simulink model "AcO_Ctrl_Geometric_headless_R2016a"  (R2016a)
settings: Solver=FixedStepDiscrete  StartTime=0.0  StopTime=simulation_duration  FixedStep=Ts  RelTol=1e-3
values from neighbouring files (symbols this model uses):
  M1_BeMo_d = zeros(7,M1_n_mode)    [AcO_Ctrl_headless_cfg.m]    (also in agws_cfg.m = 1e-6*bsxfun(@times,randn(7,M1_n_mode),scale); agws_fastTT_cfg.m = 1e-6*bsxfun(@times,randn(7,M1_n_mode),scale))
  M1_RiBo_d = zeros(7,6)    [AcO_Ctrl_headless_cfg.m]    (also in agws_cfg.m = [M1_Txyz0 M1_Rxyz0]; agws_fastTT_cfg.m = [M1_Txyz0 M1_Rxyz0])
  M2_RiBo_d = zeros(7,6)    [AcO_Ctrl_headless_cfg.m]    (also in agws_cfg.m = [M2_Txyz0 M2_Rxyz0]; agws_fastTT_cfg.m = [M2_Txyz0 M2_Rxyz0])
  Ts = 1/fs    (= 0.002)    [AcO_Ctrl_headless_cfg.m]    (also in agws_fastTT_cfg.m = 0.005)
undefined symbols (not defined in the file or in its folder): Az_C, CG2Hp, CG2Hp_S7, El_C, Fsmm, GIR_C, Hp2CG_f, Hp2CG_f_S7, HPdtf, HpK, KM2, M2_actdyn, M2_CG2Hp, M_LOS, MIMO_C, PTT2act, PTT2act_even, Q, sysd, TT2act, TT2act_even
undefined symbols (not defined in the file): on_axis_src_outputs
libraries: CEO x2
(part 6 of 6)

== system AcO_Ctrl_Geometric_headless_R2016a/Structural Dynamics V3.3/Structural Dynamics V3.5.3/Structural Dynamics Plus CL Az El M1 force/M1 Force Control/ControlM1S1/MIMO Controller ==
  In1 : Inport
  Demux1 : Demux  Outputs=6
  Gain{,1..5} (6 alike) : Gain
  Mux1 : Mux  Inputs=6
  R1 Controller : DiscreteTransferFcn  Numerator=MIMO_C(4,4).num{1}  Denominator=MIMO_C(4,4).den{1}
  R2 Controller : DiscreteTransferFcn  Numerator=MIMO_C(5,5).num{1}  Denominator=MIMO_C(5,5).den{1}
  R3 Controller : DiscreteTransferFcn  Numerator=MIMO_C(6,6).num{1}  Denominator=MIMO_C(6,6).den{1}
  T1 Controller : DiscreteTransferFcn  Numerator=MIMO_C(1,1).num{1}  Denominator=MIMO_C(1,1).den{1}
  T2 Controller : DiscreteTransferFcn  Numerator=MIMO_C(2,2).num{1}  Denominator=MIMO_C(2,2).den{1}
  T3 Controller : DiscreteTransferFcn  Numerator=MIMO_C(3,3).num{1}  Denominator=MIMO_C(3,3).den{1}
  Out1 : Outport
  wires:
  Gain5/1 -> T3 Controller/1
  Gain4/1 -> R3 Controller/1
  Gain3/1 -> R2 Controller/1
  Gain2/1 -> R1 Controller/1
  Gain1/1 -> T2 Controller/1
  Gain/1 -> T1 Controller/1
  Mux1/1 -> Out1/1
  T1 Controller/1 -> Mux1/1
  T2 Controller/1 -> Mux1/2
  T3 Controller/1 -> Mux1/3
  R1 Controller/1 -> Mux1/4
  R2 Controller/1 -> Mux1/5
  R3 Controller/1 -> Mux1/6
  Demux1/6 -> Gain4/1
  Demux1/5 -> Gain3/1
  Demux1/4 -> Gain2/1
  Demux1/3 -> Gain5/1
  Demux1/2 -> Gain1/1
  Demux1/1 -> Gain/1
  In1/1 -> Demux1/1

== system AcO_Ctrl_Geometric_headless_R2016a/Structural Dynamics V3.3/Structural Dynamics V3.5.3/Structural Dynamics Plus CL Az El M1 force/M1 Force Control/ControlM1S2/MIMO Controller ==
  In1 : Inport
  Demux1 : Demux  Outputs=6
  Gain{,1..5} (6 alike) : Gain
  Mux1 : Mux  Inputs=6
  R1 Controller : DiscreteTransferFcn  Numerator=MIMO_C(4,4).num{1}  Denominator=MIMO_C(4,4).den{1}
  R2 Controller : DiscreteTransferFcn  Numerator=MIMO_C(5,5).num{1}  Denominator=MIMO_C(5,5).den{1}
  R3 Controller : DiscreteTransferFcn  Numerator=MIMO_C(6,6).num{1}  Denominator=MIMO_C(6,6).den{1}
  T1 Controller : DiscreteTransferFcn  Numerator=MIMO_C(1,1).num{1}  Denominator=MIMO_C(1,1).den{1}
  T2 Controller : DiscreteTransferFcn  Numerator=MIMO_C(2,2).num{1}  Denominator=MIMO_C(2,2).den{1}
  T3 Controller : DiscreteTransferFcn  Numerator=MIMO_C(3,3).num{1}  Denominator=MIMO_C(3,3).den{1}
  Out1 : Outport
  wires:
  In1/1 -> Demux1/1
  Demux1/1 -> Gain/1
  Demux1/2 -> Gain1/1
  Demux1/3 -> Gain5/1
  Demux1/4 -> Gain2/1
  Demux1/5 -> Gain3/1
  Demux1/6 -> Gain4/1
  R3 Controller/1 -> Mux1/6
  R2 Controller/1 -> Mux1/5
  R1 Controller/1 -> Mux1/4
  T3 Controller/1 -> Mux1/3
  T2 Controller/1 -> Mux1/2
  T1 Controller/1 -> Mux1/1
  Mux1/1 -> Out1/1
  Gain/1 -> T1 Controller/1
  Gain1/1 -> T2 Controller/1
  Gain2/1 -> R1 Controller/1
  Gain3/1 -> R2 Controller/1
  Gain4/1 -> R3 Controller/1
  Gain5/1 -> T3 Controller/1

== system AcO_Ctrl_Geometric_headless_R2016a/Structural Dynamics V3.3/Structural Dynamics V3.5.3/Structural Dynamics Plus CL Az El M1 force/M1 Force Control/ControlM1S3/MIMO Controller ==
  In1 : Inport
  Demux1 : Demux  Outputs=6
  Gain{,1..5} (6 alike) : Gain
  Mux1 : Mux  Inputs=6
  R1 Controller : DiscreteTransferFcn  Numerator=MIMO_C(4,4).num{1}  Denominator=MIMO_C(4,4).den{1}
  R2 Controller : DiscreteTransferFcn  Numerator=MIMO_C(5,5).num{1}  Denominator=MIMO_C(5,5).den{1}
  R3 Controller : DiscreteTransferFcn  Numerator=MIMO_C(6,6).num{1}  Denominator=MIMO_C(6,6).den{1}
  T1 Controller : DiscreteTransferFcn  Numerator=MIMO_C(1,1).num{1}  Denominator=MIMO_C(1,1).den{1}
  T2 Controller : DiscreteTransferFcn  Numerator=MIMO_C(2,2).num{1}  Denominator=MIMO_C(2,2).den{1}
  T3 Controller : DiscreteTransferFcn  Numerator=MIMO_C(3,3).num{1}  Denominator=MIMO_C(3,3).den{1}
  Out1 : Outport
  wires:
  Gain5/1 -> T3 Controller/1
  Gain4/1 -> R3 Controller/1
  Gain3/1 -> R2 Controller/1
  Gain2/1 -> R1 Controller/1
  Gain1/1 -> T2 Controller/1
  Gain/1 -> T1 Controller/1
  Mux1/1 -> Out1/1
  T1 Controller/1 -> Mux1/1
  T2 Controller/1 -> Mux1/2
  T3 Controller/1 -> Mux1/3
  R1 Controller/1 -> Mux1/4
  R2 Controller/1 -> Mux1/5
  R3 Controller/1 -> Mux1/6
  Demux1/6 -> Gain4/1
  Demux1/5 -> Gain3/1
  Demux1/4 -> Gain2/1
  Demux1/3 -> Gain5/1
  Demux1/2 -> Gain1/1
  Demux1/1 -> Gain/1
  In1/1 -> Demux1/1

== system AcO_Ctrl_Geometric_headless_R2016a/Structural Dynamics V3.3/Structural Dynamics V3.5.3/Structural Dynamics Plus CL Az El M1 force/M1 Force Control/ControlM1S4/MIMO Controller ==
  In1 : Inport
  Demux1 : Demux  Outputs=6
  Gain{,1..5} (6 alike) : Gain
  Mux1 : Mux  Inputs=6
  R1 Controller : DiscreteTransferFcn  Numerator=MIMO_C(4,4).num{1}  Denominator=MIMO_C(4,4).den{1}
  R2 Controller : DiscreteTransferFcn  Numerator=MIMO_C(5,5).num{1}  Denominator=MIMO_C(5,5).den{1}
  R3 Controller : DiscreteTransferFcn  Numerator=MIMO_C(6,6).num{1}  Denominator=MIMO_C(6,6).den{1}
  T1 Controller : DiscreteTransferFcn  Numerator=MIMO_C(1,1).num{1}  Denominator=MIMO_C(1,1).den{1}
  T2 Controller : DiscreteTransferFcn  Numerator=MIMO_C(2,2).num{1}  Denominator=MIMO_C(2,2).den{1}
  T3 Controller : DiscreteTransferFcn  Numerator=MIMO_C(3,3).num{1}  Denominator=MIMO_C(3,3).den{1}
  Out1 : Outport
  wires:
  In1/1 -> Demux1/1
  Demux1/1 -> Gain/1
  Demux1/2 -> Gain1/1
  Demux1/3 -> Gain5/1
  Demux1/4 -> Gain2/1
  Demux1/5 -> Gain3/1
  Demux1/6 -> Gain4/1
  R3 Controller/1 -> Mux1/6
  R2 Controller/1 -> Mux1/5
  R1 Controller/1 -> Mux1/4
  T3 Controller/1 -> Mux1/3
  T2 Controller/1 -> Mux1/2
  T1 Controller/1 -> Mux1/1
  Mux1/1 -> Out1/1
  Gain/1 -> T1 Controller/1
  Gain1/1 -> T2 Controller/1
  Gain2/1 -> R1 Controller/1
  Gain3/1 -> R2 Controller/1
  Gain4/1 -> R3 Controller/1
  Gain5/1 -> T3 Controller/1

== system AcO_Ctrl_Geometric_headless_R2016a/Structural Dynamics V3.3/Structural Dynamics V3.5.3/Structural Dynamics Plus CL Az El M1 force/M1 Force Control/ControlM1S5/MIMO Controller ==
  In1 : Inport
  Demux1 : Demux  Outputs=6
  Gain{,1..5} (6 alike) : Gain
  Mux1 : Mux  Inputs=6
  R1 Controller : DiscreteTransferFcn  Numerator=MIMO_C(4,4).num{1}  Denominator=MIMO_C(4,4).den{1}
  R2 Controller : DiscreteTransferFcn  Numerator=MIMO_C(5,5).num{1}  Denominator=MIMO_C(5,5).den{1}
  R3 Controller : DiscreteTransferFcn  Numerator=MIMO_C(6,6).num{1}  Denominator=MIMO_C(6,6).den{1}
  T1 Controller : DiscreteTransferFcn  Numerator=MIMO_C(1,1).num{1}  Denominator=MIMO_C(1,1).den{1}
  T2 Controller : DiscreteTransferFcn  Numerator=MIMO_C(2,2).num{1}  Denominator=MIMO_C(2,2).den{1}
  T3 Controller : DiscreteTransferFcn  Numerator=MIMO_C(3,3).num{1}  Denominator=MIMO_C(3,3).den{1}
  Out1 : Outport
  wires:
  Gain5/1 -> T3 Controller/1
  Gain4/1 -> R3 Controller/1
  Gain3/1 -> R2 Controller/1
  Gain2/1 -> R1 Controller/1
  Gain1/1 -> T2 Controller/1
  Gain/1 -> T1 Controller/1
  Mux1/1 -> Out1/1
  T1 Controller/1 -> Mux1/1
  T2 Controller/1 -> Mux1/2
  T3 Controller/1 -> Mux1/3
  R1 Controller/1 -> Mux1/4
  R2 Controller/1 -> Mux1/5
  R3 Controller/1 -> Mux1/6
  Demux1/6 -> Gain4/1
  Demux1/5 -> Gain3/1
  Demux1/4 -> Gain2/1
  Demux1/3 -> Gain5/1
  Demux1/2 -> Gain1/1
  Demux1/1 -> Gain/1
  In1/1 -> Demux1/1

== system AcO_Ctrl_Geometric_headless_R2016a/Structural Dynamics V3.3/Structural Dynamics V3.5.3/Structural Dynamics Plus CL Az El M1 force/M1 Force Control/ControlM1S6/MIMO Controller ==
  In1 : Inport
  Demux1 : Demux  Outputs=6
  Gain{,1..5} (6 alike) : Gain
  Mux1 : Mux  Inputs=6
  R1 Controller : DiscreteTransferFcn  Numerator=MIMO_C(4,4).num{1}  Denominator=MIMO_C(4,4).den{1}
  R2 Controller : DiscreteTransferFcn  Numerator=MIMO_C(5,5).num{1}  Denominator=MIMO_C(5,5).den{1}
  R3 Controller : DiscreteTransferFcn  Numerator=MIMO_C(6,6).num{1}  Denominator=MIMO_C(6,6).den{1}
  T1 Controller : DiscreteTransferFcn  Numerator=MIMO_C(1,1).num{1}  Denominator=MIMO_C(1,1).den{1}
  T2 Controller : DiscreteTransferFcn  Numerator=MIMO_C(2,2).num{1}  Denominator=MIMO_C(2,2).den{1}
  T3 Controller : DiscreteTransferFcn  Numerator=MIMO_C(3,3).num{1}  Denominator=MIMO_C(3,3).den{1}
  Out1 : Outport
  wires:
  In1/1 -> Demux1/1
  Demux1/1 -> Gain/1
  Demux1/2 -> Gain1/1
  Demux1/3 -> Gain5/1
  Demux1/4 -> Gain2/1
  Demux1/5 -> Gain3/1
  Demux1/6 -> Gain4/1
  R3 Controller/1 -> Mux1/6
  R2 Controller/1 -> Mux1/5
  R1 Controller/1 -> Mux1/4
  T3 Controller/1 -> Mux1/3
  T2 Controller/1 -> Mux1/2
  T1 Controller/1 -> Mux1/1
  Mux1/1 -> Out1/1
  Gain/1 -> T1 Controller/1
  Gain1/1 -> T2 Controller/1
  Gain2/1 -> R1 Controller/1
  Gain3/1 -> R2 Controller/1
  Gain4/1 -> R3 Controller/1
  Gain5/1 -> T3 Controller/1

== system AcO_Ctrl_Geometric_headless_R2016a/Structural Dynamics V3.3/Structural Dynamics V3.5.3/Structural Dynamics Plus CL Az El M1 force/M1 Force Control/ControlM1S7/MIMO Controller ==
  In1 : Inport
  Demux1 : Demux  Outputs=6
  Gain{,1..5} (6 alike) : Gain
  Mux1 : Mux  Inputs=6
  R1 Controller : DiscreteTransferFcn  Numerator=MIMO_C(4,4).num{1}  Denominator=MIMO_C(4,4).den{1}
  R2 Controller : DiscreteTransferFcn  Numerator=MIMO_C(5,5).num{1}  Denominator=MIMO_C(5,5).den{1}
  R3 Controller : DiscreteTransferFcn  Numerator=MIMO_C(6,6).num{1}  Denominator=MIMO_C(6,6).den{1}
  T1 Controller : DiscreteTransferFcn  Numerator=MIMO_C(1,1).num{1}  Denominator=MIMO_C(1,1).den{1}
  T2 Controller : DiscreteTransferFcn  Numerator=MIMO_C(2,2).num{1}  Denominator=MIMO_C(2,2).den{1}
  T3 Controller : DiscreteTransferFcn  Numerator=MIMO_C(3,3).num{1}  Denominator=MIMO_C(3,3).den{1}
  Out1 : Outport
  wires:
  Gain5/1 -> T3 Controller/1
  Gain4/1 -> R3 Controller/1
  Gain3/1 -> R2 Controller/1
  Gain2/1 -> R1 Controller/1
  Gain1/1 -> T2 Controller/1
  Gain/1 -> T1 Controller/1
  Mux1/1 -> Out1/1
  T1 Controller/1 -> Mux1/1
  T2 Controller/1 -> Mux1/2
  T3 Controller/1 -> Mux1/3
  R1 Controller/1 -> Mux1/4
  R2 Controller/1 -> Mux1/5
  R3 Controller/1 -> Mux1/6
  Demux1/6 -> Gain4/1
  Demux1/5 -> Gain3/1
  Demux1/4 -> Gain2/1
  Demux1/3 -> Gain5/1
  Demux1/2 -> Gain1/1
  Demux1/1 -> Gain/1
  In1/1 -> Demux1/1

== matlab function AcO_Ctrl_Geometric_headless_R2016a/TT7 to M2 Rigid Body ==
  data: u input; y output
function y = TT2RiBo(u)
%#codegen

y = zeros(7,6);
y(:,4:5) = reshape(u,2,7)';

== matlab function AcO_Ctrl_Geometric_headless_R2016a/AGWS to M1 & M2 ==
  data: u input; M1RiBo output; M2RiBo output; M1BeMo output
function [M1RiBo,M2RiBo,M1BeMo] = AGWS2M12(u)
%#codegen

y = reshape(u,[],7)';
M1RiBo = y(:,[4:6,1:3]);
M2RiBo = y(:,[10:12,7:9]);
M1BeMo = y(:,13:end);

== matlab function AcO_Ctrl_Geometric_headless_R2016a/Structural Dynamics V3.3/Structural Dynamics V3.5.3/MATLAB Function ==
  data: u input; y output
function y = M2_V2M(u)
%#codegen

%y = circshift(reshape(u,6,7)',-1,1);
y = reshape(u,6,7)';

== matlab function AcO_Ctrl_Geometric_headless_R2016a/Structural Dynamics V3.3/Structural Dynamics V3.5.3/MATLAB Function1 ==
  data: u input; y output
function y = M2_V2M(u)
%#codegen

%y = circshift(reshape(u,6,7)',-1,1);
y = reshape(u,6,7)';

== matlab function AcO_Ctrl_Geometric_headless_R2016a/Structural Dynamics V3.3/Structural Dynamics V3.5.3/MATLAB Function2 ==
  data: u input; y output
function y = M1_M2V(u)
%#codegen

u = u';
y = u(:);
%y = circshift(y,6);

== matlab function AcO_Ctrl_Geometric_headless_R2016a/Structural Dynamics V3.3/Structural Dynamics V3.5.3/TT2PTT ==
  data: u input; y output
function y = fcn(u)

y = zeros(21,1);
y = reshape( u(:,3:5)', 21, 1);
%y = circshift(y,3);

== matlab function AcO_Ctrl_Geometric_headless_R2016a/Structural Dynamics V3.3/Structural Dynamics V3.3/MATLAB Function ==
  data: u input; y output
function y = M2_V2M(u)
%#codegen

y = circshift(reshape(u,6,7)',-1,1);

== matlab function AcO_Ctrl_Geometric_headless_R2016a/Structural Dynamics V3.3/Structural Dynamics V3.3/MATLAB Function1 ==
  data: u input; y output
function y = M2_V2M(u)
%#codegen

y = circshift(reshape(u,6,7)',-1,1);

== matlab function AcO_Ctrl_Geometric_headless_R2016a/Structural Dynamics V3.3/Structural Dynamics V3.3/MATLAB Function2 ==
  data: u input; y output
function y = M1_M2V(u)
%#codegen

u = u';
y = u(:);
y = circshift(y,6);

== matlab function AcO_Ctrl_Geometric_headless_R2016a/Structural Dynamics V3.3/Structural Dynamics V3.3/TT2PTT ==
  data: u input; y output
function y = fcn(u)

y = zeros(21,1);
y = reshape( u(:,3:5)', 21, 1);
y = circshift(y,3);

== matlab function AcO_Ctrl_Geometric_headless_R2016a/Structural Dynamics V3.3/Structural Dynamics V3.3a/MATLAB Function ==
  data: u input; y output
function y = M2_V2M(u)
%#codegen

y = circshift(reshape(u,6,7)',-1,1);

== matlab function AcO_Ctrl_Geometric_headless_R2016a/Structural Dynamics V3.3/Structural Dynamics V3.3a/MATLAB Function1 ==
  data: u input; y output
function y = M2_V2M(u)
%#codegen

y = circshift(reshape(u,6,7)',-1,1);

== matlab function AcO_Ctrl_Geometric_headless_R2016a/Structural Dynamics V3.3/Structural Dynamics V3.3a/MATLAB Function2 ==
  data: u input; y output
function y = M1_M2V(u)
%#codegen

u = u';
y = u(:);
y = circshift(y,6);

== matlab function AcO_Ctrl_Geometric_headless_R2016a/Structural Dynamics V3.3/Structural Dynamics V3.3a/TT2PTT ==
  data: u input; y output
function y = fcn(u)

y = zeros(21,1);
y = reshape( u(:,3:5)', 21, 1);
y = circshift(y,3);

== matlab function AcO_Ctrl_Geometric_headless_R2016a/Structural Dynamics V3.3/Structural Dynamics V3.1/M1 Segments/MATLAB Function ==
  data: u input; s7 output; s1 output; s2 output; s3 output; s4 output; s5 output; s6 output
function [s7,s1,s2,s3,s4,s5,s6] = M1_M2V(u)
%#codegen

u = u';
s7 = u(:,7);
s1 = u(:,1);
s2 = u(:,2);
s3 = u(:,3);
s4 = u(:,4);
s5 = u(:,5);
s6 = u(:,6);

== matlab function AcO_Ctrl_Geometric_headless_R2016a/Structural Dynamics V3.3/Structural Dynamics V3.1/MATLAB Function ==
  data: u input; y output
function y = M2_V2M(u)
%#codegen

y = circshift(reshape(u,6,7)',-1,1);

== matlab function AcO_Ctrl_Geometric_headless_R2016a/Structural Dynamics V3.3/Structural Dynamics V3.1/MATLAB Function1 ==
  data: u input; s7 output; s1 output; s2 output; s3 output; s4 output; s5 output; s6 output
function [s7,s1,s2,s3,s4,s5,s6] = M2_DOF2TT(u)
%#codegen

u = u';
s7 = u(4:5,7);
s1 = u(4:5,1);
s2 = u(4:5,2);
s3 = u(4:5,3);
s4 = u(4:5,4);
s5 = u(4:5,5);
s6 = u(4:5,6);

== matlab function AcO_Ctrl_Geometric_headless_R2016a/Structural Dynamics V3.3/Structural Dynamics V3.1/MATLAB Function2 ==
  data: u input; y output
function y = M2_V2M(u)
%#codegen


y = circshift(reshape(u,6,7)',-1,1);

== matlab function AcO_Ctrl_Geometric_headless_R2016a/Structural Dynamics V3.3/Structural Dynamics V3.5.2/MATLAB Function ==
  data: u input; y output
function y = M2_V2M(u)
%#codegen

y = circshift(reshape(u,6,7)',-1,1);

== matlab function AcO_Ctrl_Geometric_headless_R2016a/Structural Dynamics V3.3/Structural Dynamics V3.5.2/MATLAB Function1 ==
  data: u input; y output
function y = M2_V2M(u)
%#codegen

y = circshift(reshape(u,6,7)',-1,1);

== matlab function AcO_Ctrl_Geometric_headless_R2016a/Structural Dynamics V3.3/Structural Dynamics V3.5.2/MATLAB Function2 ==
  data: u input; y output
function y = M1_M2V(u)
%#codegen

u = u';
y = u(:);
y = circshift(y,6);

== matlab function AcO_Ctrl_Geometric_headless_R2016a/Structural Dynamics V3.3/Structural Dynamics V3.5.2/TT2PTT ==
  data: u input; y output
function y = fcn(u)

y = zeros(21,1);
y = reshape( u(:,3:5)', 21, 1);
y = circshift(y,3);
